simulink model "algebraic_constraint9_1"  (Simulink 7.3)
settings: Solver=VariableStepDiscrete  StartTime=0.0  StopTime=10.0  MaxStep=0.1  RelTol=1e-3
libraries: simulink x2
settings Model: Creator=sn00632  LastModifiedBy=sn00632
settings DebuggingCC: AlgebraicLoopMsg=none  ArtificialAlgebraicLoopMsg=none

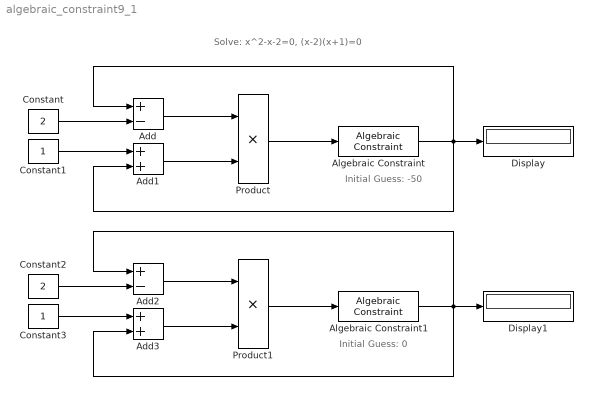
== system algebraic_constraint9_1 ==
  note: Solve: x^2-x-2=0, (x-2)(x+1)=0
  note: Initial Guess: -50
  note: Initial Guess: 0
  Add : Sum  Inputs=+-  OutDataType=fixdt(1, 16)  OutScaling=2^-10
  Add1 : Sum  OutDataType=fixdt(1, 16)  OutScaling=2^-10
  Add2 : Sum  Inputs=+-  OutDataType=fixdt(1, 16)  OutScaling=2^-10
  Add3 : Sum  OutDataType=fixdt(1, 16)  OutScaling=2^-10
  Algebraic Constraint : simulink/Math Operations/Algebraic Constraint  SystemSampleTime=-1  z0=-50
  Algebraic Constraint1 : simulink/Math Operations/Algebraic Constraint  SystemSampleTime=-1  z0=0
  Constant : Constant  Value=2  OutDataType=fixdt(1, 16)  OutScaling=2^0
  Constant1 : Constant  OutDataType=fixdt(1, 16)  OutScaling=2^0
  Constant2 : Constant  Value=2  OutDataType=fixdt(1, 16)  OutScaling=2^0
  Constant3 : Constant  OutDataType=fixdt(1, 16)  OutScaling=2^0
  Display : Display
  Display1 : Display
  Product : Product  OutDataType=fixdt(1, 16)  OutScaling=2^0  RndMeth=Zero
  Product1 : Product  OutDataType=fixdt(1, 16)  OutScaling=2^0  RndMeth=Zero
  wires:
  Product/1 -> Algebraic Constraint/1
  Algebraic Constraint/1 -> Display/1, Add1/2, Add/1
  Add/1 -> Product/1
  Add1/1 -> Product/2
  Constant/1 -> Add/2
  Constant1/1 -> Add1/1
  Product1/1 -> Algebraic Constraint1/1
  Algebraic Constraint1/1 -> Add2/1, Add3/2, Display1/1
  Add2/1 -> Product1/1
  Add3/1 -> Product1/2
  Constant2/1 -> Add2/2
  Constant3/1 -> Add3/1
